simulink model "model_1d"  (R2018b)
settings: Solver=VariableStepAuto  StartTime=0.0  StopTime=10  RelTol=1e-3
settings Model: Creator=valeriiche  LastModifiedBy=valeriiche

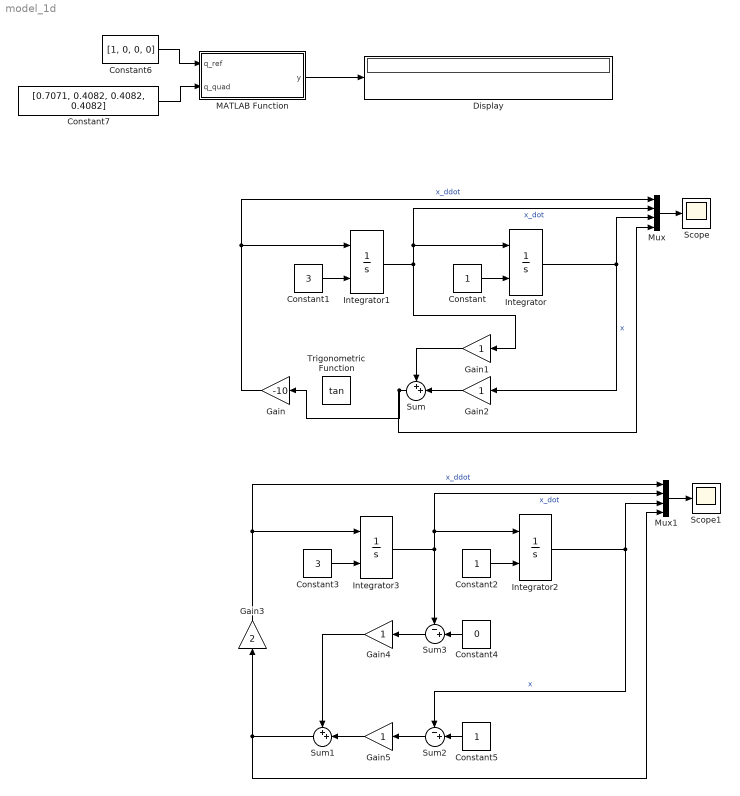
== system model_1d ==
  Constant : Constant
  Constant1 : Constant  Value=3
  Constant2 : Constant
  Constant3 : Constant  Value=3
  Constant4 : Constant  Value=0
  Constant5 : Constant
  Constant6 : Constant  Value=[1, 0, 0, 0]
  Constant7 : Constant  Value=[0.7071, 0.4082, 0.4082, 0.4082]
  Display : Display
  Gain : Gain  Gain=-10
  Gain{1..2,4..5} (4 alike) : Gain
  Gain3 : Gain  Gain=2
  Integrator{,1..3} (4 alike) : Integrator  InitialConditionSource=external
  MATLAB Function : MATLAB Function  TreatAsAtomicUnit=on
  Mux : Mux
  Mux1 : Mux
  Scope : Scope
  Scope1 : Scope
  Sum : Sum  Inputs=++|
  Sum1 : Sum  Inputs=++|
  Sum2 : Sum  Inputs=-+|
  Sum3 : Sum  Inputs=-+|
  Trigonometric Function : Trigonometry  Operator=tan
  wires:
  Mux/1 -> Scope/1
  Constant/1 -> Integrator/2
  Constant1/1 -> Integrator1/2
  Integrator1/1 -> Gain1/1, Integrator/1, Mux/2  "x_dot"
  Gain/1 -> Integrator1/1, Mux/1  "x_ddot"
  Integrator/1 -> Mux/3, Gain2/1  "x"
  Gain2/1 -> Sum/2
  Gain1/1 -> Sum/1
  Sum/1 -> Gain/1, Mux/4
  Constant2/1 -> Integrator2/2
  Sum1/1 -> Gain3/1, Mux1/4
  Mux1/1 -> Scope1/1
  Integrator3/1 -> Mux1/2, Integrator2/1, Sum3/1  "x_dot"
  Gain5/1 -> Sum1/2
  Gain3/1 -> Integrator3/1, Mux1/1  "x_ddot"
  Integrator2/1 -> Mux1/3, Sum2/1  "x"
  Constant3/1 -> Integrator3/2
  Gain4/1 -> Sum1/1
  Sum2/1 -> Gain5/1
  Sum3/1 -> Gain4/1
  Constant4/1 -> Sum3/2
  Constant5/1 -> Sum2/2
  Constant6/1 -> MATLAB Function/1(q_ref)
  Constant7/1 -> MATLAB Function/2(q_quad)
  MATLAB Function/1(y) -> Display/1

== matlab function model_1d/MATLAB Function ==
  data: q_ref input; y output; q_quad input
function y = fcn(q_ref, q_quad)

q_quad_conj = [ q_quad(1), -q_quad(2), -q_quad(3), -q_quad(4) ];

y = [[ q_ref(1), -q_ref(2), -q_ref(3), -q_ref(4)];
     [ q_ref(2),  q_ref(1), -q_ref(4),  q_ref(3)];
     [ q_ref(3),  q_ref(4),  q_ref(1), -q_ref(2)];
     [ q_ref(4), -q_ref(3),  q_ref(2),  q_ref(1)]] * q_quad_conj';

% y = quat_multiply(q_ref, quat_conjugate(q_quad));
